simulink model "untitled1"  (R2024b)
settings: Solver=VariableStepAuto  StartTime=0.0  StopTime=10.0  RelTol=1e-3
settings Model: Creator=C27Lucan.Keyser  LastModifiedBy=C27Lucan.Keyser

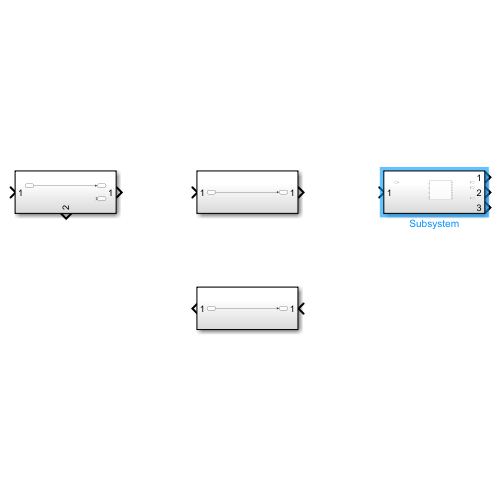
[thumbnail: Simulink's stored preview of the top-level diagram]
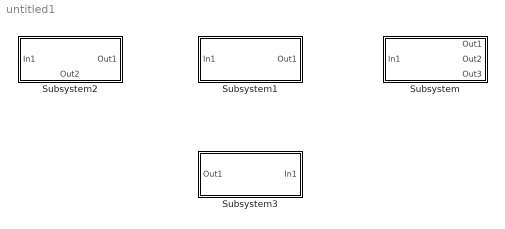
== system untitled1 ==
  Subsystem : Subsystem
  Subsystem1 : Subsystem
  Subsystem2 : Subsystem
      settings: PortSchema="{\"entries\":[{\"content\":{\"sides\":[{\"content\":{\"connectorIds\":[\"In1\"]},\"type\":\"ConnectorPlacement.EquallySpacedRectSide\",\"uuid\":\"1679087d-7353-4f43-848c-bb56766678c5\"},{\"content\":{\"connectorIds\":[\"Out1\"],\"side\":\"RIGHT\"},\"type\":\"ConnectorPlacement.EquallySpacedRectSide\",\"uuid\":\"e5745018-1815-4126-8f7b-43368347b77a\"},{\"content\":{\"side\":\"TOP\"},\"type\":\"ConnectorPlacement.EquallySpacedRectSide\",\"uuid\":\"bc3432ca-3ef8-4ef0-a14e-d9e37ebacf89\"},{\"content\":{\"connectorIds\":[\"Out2\"],\"side\":\"BOTTOM\"},\"type\":\"ConnectorPlacement.EquallySpacedRectSide\",\"uuid\":\"426457a8-8c63-4a9e-9613-e80617fb969c\"}]},\"type\":\"ConnectorPlacement.EquallySpacedConnector\",\"uuid\":\"08651911-01d4-4f33-87f1-6b92b7c4679f\"}],\"packageUris\":[\"http://schema.mathworks.com/mf0/Connector/R2020b\"],\"version\":\"1.0\"}"
  Subsystem3 : Subsystem

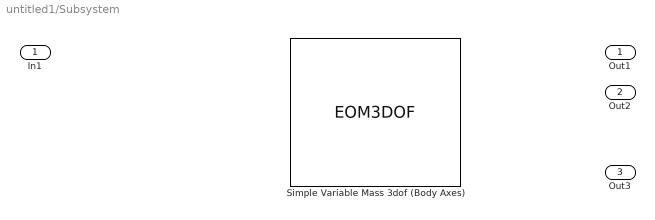
== system untitled1/Subsystem ==
  In1 : Inport
  Simple Variable Mass 3dof (Body Axes) : EOM3DOF  mtype=Simple Variable
  Out1 : Outport
  Out2 : Outport  Port=2
  Out3 : Outport  Port=3

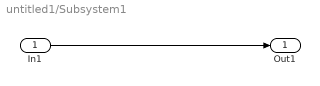
== system untitled1/Subsystem1 ==
  In1 : Inport
  Out1 : Outport
  wires:
  In1/1 -> Out1/1

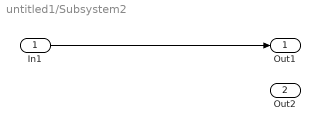
== system untitled1/Subsystem2 ==
  In1 : Inport
  Out1 : Outport
  Out2 : Outport  Port=2
  wires:
  In1/1 -> Out1/1

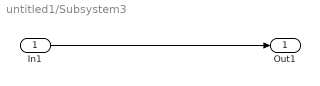
== system untitled1/Subsystem3 ==
  In1 : Inport
  Out1 : Outport
  wires:
  In1/1 -> Out1/1
